simulink model "WholeModelPIDAntiWindupDigital"  (R2020b)
settings: Solver=ode45  StartTime=0.0  StopTime=5  RelTol=1e-3
settings Model: Creator=umberto  LastModifiedBy=umbe

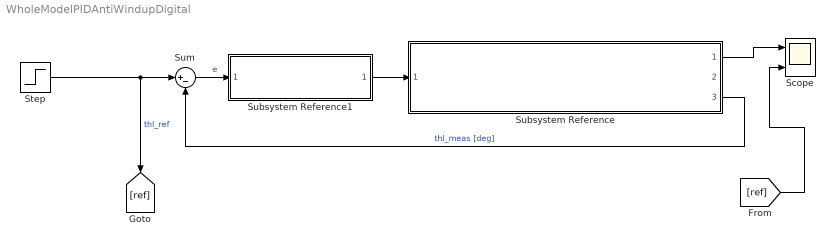
== system WholeModelPIDAntiWindupDigital ==
  Scope : Scope  NumInputPorts=2
  Step : Step  Time=0  After=70  SampleTime=0
  Subsystem Reference : Subsystem  ReferencedSubsystem=DCServoMotor_SubSystem
  Subsystem Reference1 : Subsystem  ReferencedSubsystem=PIDAntiWindupDigital_SubSystem
  Sum : Sum  Inputs=|+-
  wires:
  Subsystem Reference/3 -> Sum/2  "thl_meas [deg]"
  Step/1 -> [ref], Sum/1  "thl_ref"
  Subsystem Reference/1 -> Scope/1
  Sum/1 -> Subsystem Reference1/1  "e"
  [ref] -> Scope/2
  Subsystem Reference1/1 -> Subsystem Reference/1
